simulink model "modulation_AM"  (R2020a)
settings: Solver=VariableStepAuto  StartTime=0.0  StopTime=10  RelTol=1e-3
libraries: dsparch4 x1
settings Model: Creator=kiril_000  LastModifiedBy=kiril_000

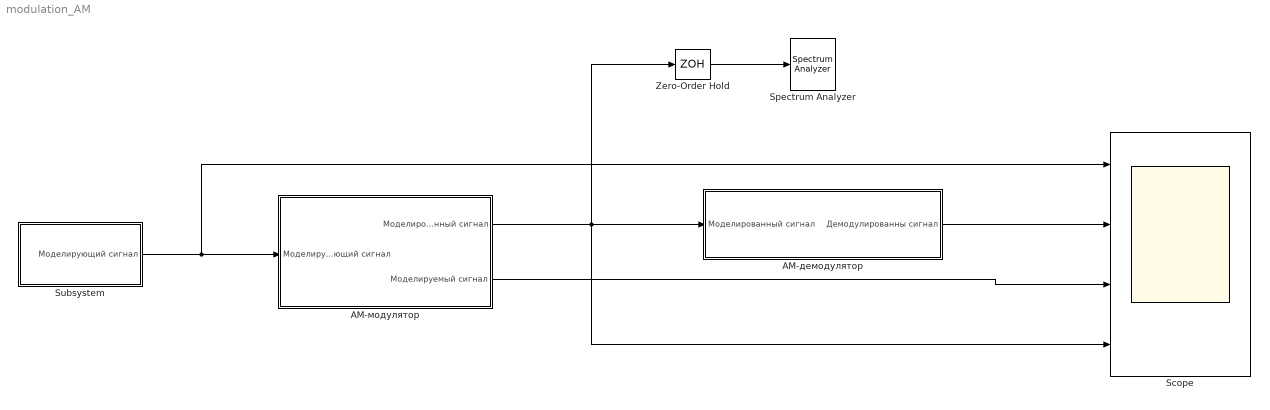
== system modulation_AM ==
  AM-демодулятор : Subsystem  mask{omega_p=1000}
      mask prompts: omega_p "Частота приёмника"
  AM-модулятор : Subsystem  mask{m=0.7, omega=1000}
      mask prompts: m "Порядок AM-модуляции"; omega "Частота несущей"
  Scope : Scope  NumInputPorts=4
  Spectrum Analyzer : SpectrumAnalyzer
  Subsystem : Subsystem
  Zero-Order Hold : ZeroOrderHold  SampleTime=1/5000
  wires:
  Subsystem/1(Моделирующий сигнал) -> Scope/1, AM-модулятор/1(Моделирующий сигнал)
  AM-модулятор/1(Моделированный сигнал) -> Zero-Order Hold/1, Scope/4, AM-демодулятор/1(Моделированный сигнал)
  AM-демодулятор/1(Демодулированны сигнал) -> Scope/2
  AM-модулятор/2(Моделируемый сигнал) -> Scope/3
  Zero-Order Hold/1 -> Spectrum Analyzer/1

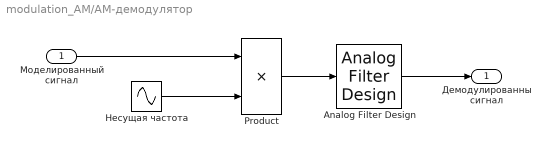
== system modulation_AM/AM-демодулятор ==
  Моделированный сигнал : Inport
  Analog Filter Design : dsparch4/Analog Filter Design  method=Butterworth  filttype=Lowpass  N=16  Wlo=2*pi*1200  Whi=80  Rp=2  Rs=40
  Product : Product
  Несущая частота : Sin  Frequency=2*pi*omega_p  SampleTime=0
  Демодулированны сигнал : Outport
  wires:
  Моделированный сигнал/1 -> Product/1
  Несущая частота/1 -> Product/2
  Analog Filter Design/1 -> Демодулированны сигнал/1
  Product/1 -> Analog Filter Design/1

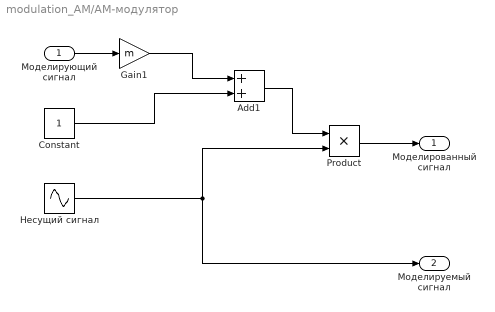
== system modulation_AM/AM-модулятор ==
  Моделирующий сигнал : Inport
  Add1 : Sum
  Constant : Constant
  Gain1 : Gain  Gain=m
  Product : Product
  Несущий сигнал : Sin  Frequency=2*pi*omega  SampleTime=0
  Моделированный сигнал : Outport
  Моделируемый сигнал : Outport  Port=2
  wires:
  Constant/1 -> Add1/2
  Gain1/1 -> Add1/1
  Add1/1 -> Product/1
  Product/1 -> Моделированный сигнал/1
  Моделирующий сигнал/1 -> Gain1/1
  Несущий сигнал/1 -> Моделируемый сигнал/1, Product/2

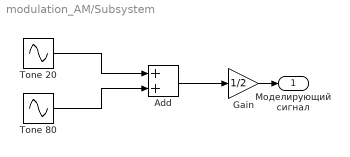
== system modulation_AM/Subsystem ==
  Add : Sum
  Gain : Gain  Gain=1/2
  Tone 20 : Sin  Frequency=2*pi*20  SampleTime=0
  Tone 80 : Sin  Frequency=2*pi*80  SampleTime=0
  Моделирующий сигнал : Outport
  wires:
  Add/1 -> Gain/1
  Tone 80/1 -> Add/2
  Gain/1 -> Моделирующий сигнал/1
  Tone 20/1 -> Add/1
